simulink model "ex4_1"  (R2015a)
settings: Solver=ode23t  StartTime=0.0  StopTime=0.1  MaxStep=1e-5  RelTol=1e-4
undefined symbols (not defined in the file): jsin
libraries: powerlib x1
settings Model: CovHtmlReporting=off  Creator=hi  LastModifiedBy=Omid
settings DataIOCC: SaveFormat=Dataset
settings HardwareCC: ProdBitPerPointer=64  ProdLargestAtomicFloat=Float  ProdIntDivRoundTo=Zero  ProdEndianess=LittleEndian  ProdHWDeviceType=Specified
settings SimscapeCC: SimscapeNormalizeSystem=off

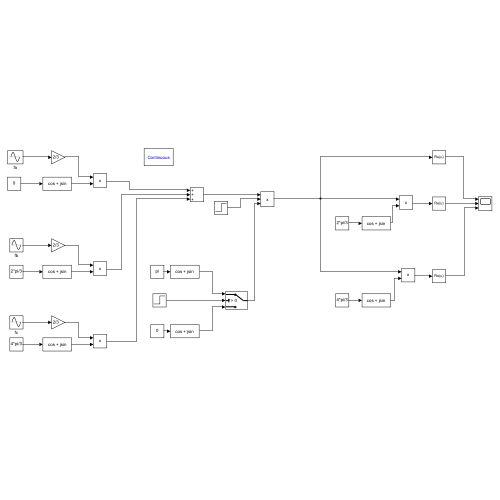
[thumbnail: Simulink's stored preview of the top-level diagram]
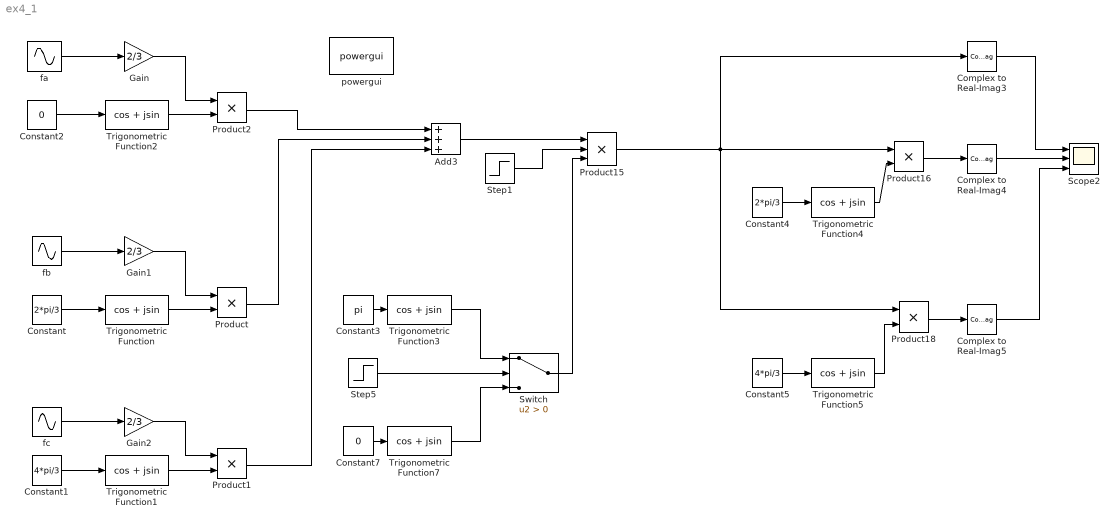
== system ex4_1 ==
  Add3 : Sum  Inputs=+++
  Complex to Real-Imag3 : ComplexToRealImag  Output=Real
  Complex to Real-Imag4 : ComplexToRealImag  Output=Real
  Complex to Real-Imag5 : ComplexToRealImag  Output=Real
  Constant : Constant  Value=2*pi/3
  Constant1 : Constant  Value=4*pi/3
  Constant2 : Constant  Value=0
  Constant3 : Constant  Value=pi
  Constant4 : Constant  Value=2*pi/3
  Constant5 : Constant  Value=4*pi/3
  Constant7 : Constant  Value=0
  Gain : Gain  Gain=2/3
  Gain1 : Gain  Gain=2/3
  Gain2 : Gain  Gain=2/3
  Product{,1..2,16,18} (5 alike) : Product
  Product15 : Product  Inputs=3
  Scope2 : Scope  NumInputPorts=3
      settings: TimeRange=auto  MaxDataPoints=5000  SaveToWorkspace=off  YMin=-2.8125~-5~-5  YMax=2.8125~5~5  SampleTime=-1
  Step1 : Step  Time=0.066  Before=1  After=1.5  SampleTime=0
  Step5 : Step  Time=0.018  SampleTime=0
  Switch : Switch  Criteria=u2 > Threshold
  Trigonometric Function{,1..5,7} (7 alike) : Trigonometry  Operator=cos + jsin
  fa : Sin  Frequency=377  Phase=pi/2  SampleTime=0
  fb : Sin  Frequency=377  Phase=-2*pi/3+pi/2  SampleTime=0
  fc : Sin  Frequency=377  Phase=-4*pi/3+pi/2  SampleTime=0
  powergui : powerlib/powergui  Priority=1  SimulationMode=Continuous  SampleTime=50e-6  frequency=60  Iterations=50  frequencyindice=60  Pbase=100e6  ErrMax=1e-4  UnitsV=kV  UnitsW=MW  buscounter=0  FunctionMessages=off  echomessages=off  EnableUseOfTLC=off  CurrentSourceSwitches=on  DisableSnubberDevices=off  DisableRonSwitches=off  DisableVfSwitches=off  DisplayEquations=off  AutomaticDiscreteSolvers=off  SolverType=Tustin/Backward Euler (TBE)  Interpol=off  ExternalGateDelay=off  methode=off  Ts=10  x0status=blocks  SPID=off  SwTol=0  HookPort=off  NonlinearTolerance=1e-4  nMaxIteration=100  ContinueOnMaxIteration=off  RestoreLinks=warning  ResistiveCurrentMeasurement=off  Frange=[0:2:500]  Ylog=off  Xlog=on  ShowGrid=off  save=off  variable=ZData  structure=0  ZoomFFT=off  StartTime=0.0  cycles=1  DisplayStyle=1  fundamental=60  FreqAxis=off  MaxFrequency=1000  frequencyindicesteady=1  RmsSteady=1  display=off
  wires:
  Constant/1 -> Trigonometric Function/1
  Trigonometric Function/1 -> Product/2
  Trigonometric Function1/1 -> Product1/2
  Constant1/1 -> Trigonometric Function1/1
  fc/1 -> Gain2/1
  fb/1 -> Gain1/1
  Constant2/1 -> Trigonometric Function2/1
  Trigonometric Function2/1 -> Product2/2
  fa/1 -> Gain/1
  Product2/1 -> Add3/1
  Product/1 -> Add3/2
  Product1/1 -> Add3/3
  Add3/1 -> Product15/1
  Step1/1 -> Product15/2
  Constant3/1 -> Trigonometric Function3/1
  Step5/1 -> Switch/2
  Constant4/1 -> Trigonometric Function4/1
  Constant5/1 -> Trigonometric Function5/1
  Product15/1 -> Complex to Real-Imag3/1, Product18/1, Product16/1
  Trigonometric Function4/1 -> Product16/2
  Trigonometric Function5/1 -> Product18/2
  Product16/1 -> Complex to Real-Imag4/1
  Product18/1 -> Complex to Real-Imag5/1
  Complex to Real-Imag4/1 -> Scope2/2
  Complex to Real-Imag3/1 -> Scope2/1
  Complex to Real-Imag5/1 -> Scope2/3
  Trigonometric Function3/1 -> Switch/1
  Trigonometric Function7/1 -> Switch/3
  Constant7/1 -> Trigonometric Function7/1
  Switch/1 -> Product15/3
  Gain/1 -> Product2/1
  Gain1/1 -> Product/1
  Gain2/1 -> Product1/1
